simulink model "STEMOLITION_V4_TWOARMCLAW_V1"  (R2021a)
settings: Solver=FixedStepAuto  StartTime=0.0  StopTime=inf  RelTol=1e-3
libraries: vexarmcortexlib x25, vexcommonlib x7
settings Model: ExtModeTrigDuration=25  Creator=nicoa  LastModifiedBy=Mihai Nicoara
settings SolverCC: AlgebraicLoopSolver=TrustRegion
settings OptimizationCC: EnhancedBackFolding=on  PassReuseOutputArgsAs=Individual arguments  ZeroExternalMemoryAtStartup=off  ZeroInternalMemoryAtStartup=off  MaxStackSize=64  OptimizeBlockOrder=speed  DifferentSizesBufferReuse=on  OptimizationCustomize=off  EfficientTunableParamExpr=on
settings DebuggingCC: ParameterTunabilityLossMsg=error  SFMachineParentedDataDiag=warning
settings HardwareCC: ProdBitPerPointer=32  ProdBitPerSizeT=32  ProdBitPerPtrDiffT=32  ProdLargestAtomicInteger=Long  ProdLargestAtomicFloat=Double  ProdWordSize=32  ProdHWDeviceType=ARM Compatible->ARM Cortex
settings SFSimCC: MATLABDynamicMemAlloc=off
settings RTWCC: SystemTargetFile=ert.tlc  HardwareBoard=ARM Cortex-based VEX Microcontroller  TLCOptions="-aInlineSetEventsForThisBaseRateFcn=TLC_FALSE -aSuppressMultiTaskScheduler=TLC_FALSE  -aRateBasedStepFcn=0"  TemplateMakefile=ert_default_tmf  GenerateReport=on  Toolchain=GNU Tools for VEX ARM Cortex  IncludeHyperlinkInReport=on  LaunchReport=on  GenerateTraceInfo=on  GenerateTraceReport=on  GenerateTraceReportSl=on  GenerateTraceReportSf=on  GenerateTraceReportEml=on
settings CodeAppCC: ForceParamTrailComments=on  IgnoreCustomStorageClasses=off  OperatorAnnotations=on  SimulinkDataObjDesc=on  SFDataObjDesc=on  InsertBlockDesc=on

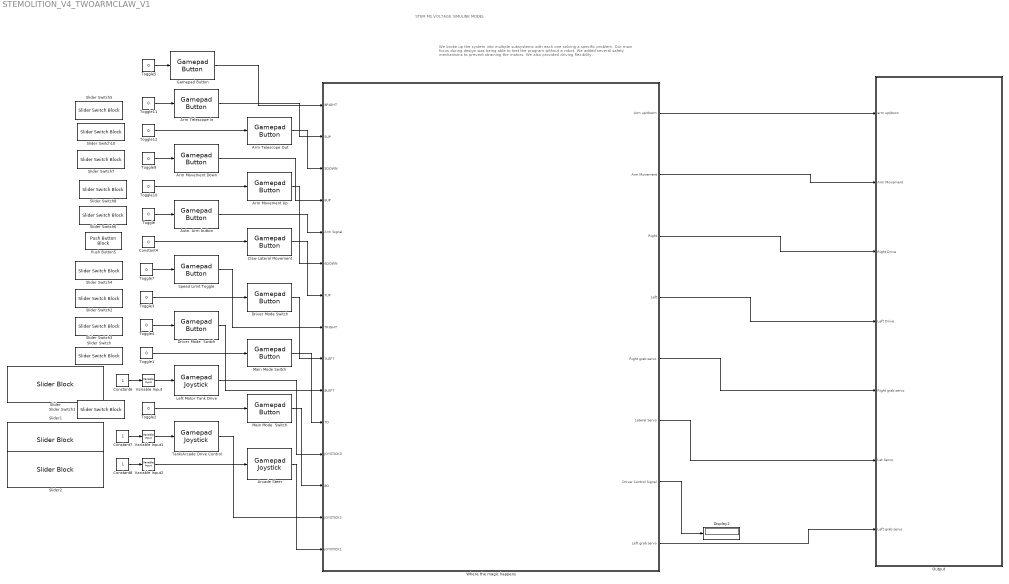
== system STEMOLITION_V4_TWOARMCLAW_V1 ==
  note: We broke up the system into multiple subsystems with each one solving a specific problem. Our main focus during
      | design was being able to test the program without a robot. We added several safety mechanisms to prevent straining
      |  the motors. We also provided driving flexibility.
  note: STEM MS VOLTAGE SIMULINK MODEL
  "Arcade Steer " : vexarmcortexlib/Gamepad/Gamepad Joystick  joystick=1  chan=1  SimulationIn=on  SampleTime=0.02
      settings: SourceProductBaseCode=EC_VEX_MICRO
  Arm Movement Down : vexarmcortexlib/Gamepad/Gamepad Button  joystick=1  chan=6  button56=Down  button78=Down  SimulationIn=on  SampleTime=0.02
      settings: SourceProductBaseCode=EC_VEX_MICRO
  Arm Movement Up : vexarmcortexlib/Gamepad/Gamepad Button  joystick=1  chan=6  button56=Up  button78=Down  SimulationIn=on  SampleTime=0.02
      settings: SourceProductBaseCode=EC_VEX_MICRO
  Arm Telescope In : vexarmcortexlib/Gamepad/Gamepad Button  joystick=1  chan=5  button56=Down  button78=Down  SimulationIn=on  SampleTime=0.02
      settings: SourceProductBaseCode=EC_VEX_MICRO
  Arm Telescope Out : vexarmcortexlib/Gamepad/Gamepad Button  joystick=1  chan=5  button56=Up  button78=Down  SimulationIn=on  SampleTime=0.02
      settings: SourceProductBaseCode=EC_VEX_MICRO
  Auto. Arm button : vexarmcortexlib/Gamepad/Gamepad Button  joystick=1  chan=8  button56=Up  button78=Up  SimulationIn=on  SampleTime=0.02
      settings: SourceProductBaseCode=EC_VEX_MICRO
  Claw Lateral Movement : vexarmcortexlib/Gamepad/Gamepad Button  joystick=1  chan=7  button56=Up  button78=Up  SimulationIn=on  SampleTime=0.02
      settings: SourceProductBaseCode=EC_VEX_MICRO
  Constant4 : Constant  Value=0
  Constant6 : Constant
  Constant7 : Constant
  Constant8 : Constant
  Display2 : Display
  Driver Mode  Switch : vexarmcortexlib/Gamepad/Gamepad Button  joystick=1  chan=8  button56=Up  button78=Left  SimulationIn=on  SampleTime=0.02
      settings: SourceProductBaseCode=EC_VEX_MICRO
  Driver Mode Switch : vexarmcortexlib/Gamepad/Gamepad Button  joystick=1  chan=7  button56=Up  button78=Left  SimulationIn=on  SampleTime=0.02
      settings: SourceProductBaseCode=EC_VEX_MICRO
  Gamepad Button : vexarmcortexlib/Gamepad/Gamepad Button  joystick=1  chan=8  button56=Up  button78=Right  SimulationIn=on  SampleTime=0.02
      settings: SourceProductBaseCode=EC_VEX_MICRO
  Left Motor Tank Drive : vexarmcortexlib/Gamepad/Gamepad Joystick  joystick=1  chan=3  SimulationIn=on  SampleTime=0.02
      settings: SourceProductBaseCode=EC_VEX_MICRO
  Main Mode  Switch : vexarmcortexlib/Gamepad/Gamepad Button  joystick=1  chan=8  button56=Up  button78=Down  SimulationIn=on  SampleTime=0.02
      settings: SourceProductBaseCode=EC_VEX_MICRO
  Main Mode Switch : vexarmcortexlib/Gamepad/Gamepad Button  joystick=1  chan=7  button56=Up  button78=Down  SimulationIn=on  SampleTime=0.02
      settings: SourceProductBaseCode=EC_VEX_MICRO
  Output : Subsystem
  Push Button5 : PushButtonBlock
  Slider : SliderBlock  LabelPosition=Hide  ScaleMin=-127  ScaleMax=127
  Slider Switch{,1..5,7..8,10} (9 alike) : SliderSwitchBlock  LabelPosition=Hide
      settings: Values={{'Off', 'On'}, [0 1]}
  Slider Switch6 : SliderSwitchBlock
      settings: Values={{'Off', 'On'}, [0 1]}
  Slider1 : SliderBlock  LabelPosition=Hide  ScaleMin=-127  ScaleMax=127
  Slider2 : SliderBlock  LabelPosition=Hide  ScaleMin=-127  ScaleMax=127
  Speed Limit Toggle : vexarmcortexlib/Gamepad/Gamepad Button  joystick=1  chan=7  button56=Up  button78=Right  SimulationIn=on  SampleTime=0.02
      settings: SourceProductBaseCode=EC_VEX_MICRO
  Tank/Arcade Drive Control : vexarmcortexlib/Gamepad/Gamepad Joystick  joystick=1  chan=2  SimulationIn=on  SampleTime=0.02
      settings: SourceProductBaseCode=EC_VEX_MICRO
  Toggle{,1..5,7,9..12} (11 alike) : Constant  Value=0
      settings: OpenFcn=|
      | if strcmp('0',get_param(gcb, 'Value'))                        set_param(gcb, 'Value', '1');
      | else
      |             set_param(gcb, 'Value', '0');
      | end
  Variable Input : vexarmcortexlib/Utilities/Variable Input  low=-127  gain=-29.69085144927537  high=127
      settings: SourceProductBaseCode=EC_VEX_MICRO
  Variable Input1 : vexarmcortexlib/Utilities/Variable Input  low=-127  gain=0  high=127
      settings: SourceProductBaseCode=EC_VEX_MICRO
  Variable Input2 : vexarmcortexlib/Utilities/Variable Input  low=-127  gain=0  high=127
      settings: SourceProductBaseCode=EC_VEX_MICRO
  Where the magic happens : Subsystem
  wires:
  Main Mode  Switch/1 -> Where the magic happens/13(8D)
  Main Mode Switch/1 -> Where the magic happens/11(7D)
  Driver Mode  Switch/1 -> Where the magic happens/10(8LEFT)
  Driver Mode Switch/1 -> Where the magic happens/9(7LEFT)
  Speed Limit Toggle/1 -> Where the magic happens/8(7RIGHT)
  Tank/Arcade Drive Control/1 -> Where the magic happens/14(JOYSTICK2)
  Left Motor Tank Drive/1 -> Where the magic happens/12(JOYSTICK3)
  "Arcade Steer "/1 -> Where the magic happens/15(JOYSTICK1)
  Claw Lateral Movement/1 -> Where the magic happens/7(7UP)
  Arm Movement Up/1 -> Where the magic happens/6(6DOWN)
  Arm Movement Down/1 -> Where the magic happens/4(6UP)
  Arm Telescope Out/1 -> Where the magic happens/3(5DOWN)
  Arm Telescope In/1 -> Where the magic happens/2(5UP)
  Toggle11/1 -> Arm Telescope In/1
  Toggle12/1 -> Arm Telescope Out/1
  Toggle9/1 -> Arm Movement Down/1
  Toggle10/1 -> Arm Movement Up/1
  Constant4/1 -> Claw Lateral Movement/1
  Toggle7/1 -> Speed Limit Toggle/1
  Toggle4/1 -> Driver Mode  Switch/1
  Toggle1/1 -> Main Mode Switch/1
  Constant6/1 -> Variable Input/1
  Variable Input/1 -> Left Motor Tank Drive/1
  Variable Input1/1 -> Tank/Arcade Drive Control/1
  Constant7/1 -> Variable Input1/1
  Variable Input2/1 -> "Arcade Steer "/1
  Constant8/1 -> Variable Input2/1
  Toggle2/1 -> Main Mode  Switch/1
  Toggle3/1 -> Driver Mode Switch/1
  Where the magic happens/7(Driver Control Signal) -> Display2/1
  Where the magic happens/6(Lateral Servo) -> Output/6(Lat Servo)
  Where the magic happens/5(Right grab servo) -> Output/5(Right grab servo)
  Where the magic happens/1(Arm up/dowm) -> Output/1(arm up/down)
  Where the magic happens/2(Arm Movement) -> Output/2(Arm Movement)
  Toggle5/1 -> Gamepad Button/1
  Gamepad Button/1 -> Where the magic happens/1(8RIGHT)
  Where the magic happens/3(Right) -> Output/3(Right Drive)
  Where the magic happens/4(Left) -> Output/4(Left Drive)
  Auto. Arm button/1 -> Where the magic happens/5(Arm Signal)
  Toggle/1 -> Auto. Arm button/1
  Where the magic happens/8(Left grab servo) -> Output/7(Left grab servo)

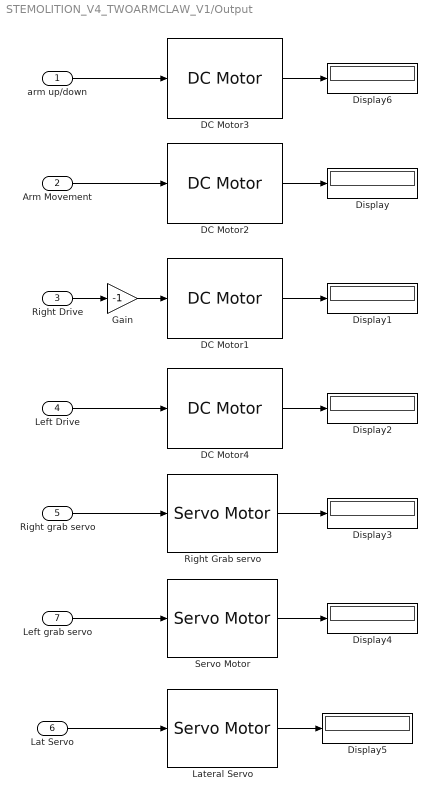
== system STEMOLITION_V4_TWOARMCLAW_V1/Output ==
  arm up/down : Inport
  Arm Movement : Inport  Port=2
  Right Drive : Inport  Port=3
  Left Drive : Inport  Port=4
  Right grab servo : Inport  Port=5
  Lat Servo : Inport  Port=6
  Left grab servo : Inport  Port=7
  DC Motor1 : vexarmcortexlib/Actuators/DC Motor  motor=2  scaleFactor=1/13.5  SimulationOut=on
      settings: SourceProductBaseCode=EC_VEX_MICRO
  DC Motor2 : vexarmcortexlib/Actuators/DC Motor  motor=4  scaleFactor=1/13.5  SimulationOut=on
      settings: SourceProductBaseCode=EC_VEX_MICRO
  DC Motor3 : vexarmcortexlib/Actuators/DC Motor  motor=7  scaleFactor=1/13.5  SimulationOut=on
      settings: SourceProductBaseCode=EC_VEX_MICRO
  DC Motor4 : vexarmcortexlib/Actuators/DC Motor  motor=9  scaleFactor=1/13.5  SimulationOut=on
      settings: SourceProductBaseCode=EC_VEX_MICRO
  Display{,1..6} (7 alike) : Display
  Gain : Gain  Gain=-1
  Lateral Servo : vexarmcortexlib/Actuators/Servo Motor  motor=8  scaleFactor=60/127  SimulationOut=on
      settings: SourceProductBaseCode=EC_VEX_MICRO
  Right Grab servo : vexarmcortexlib/Actuators/Servo Motor  motor=3  scaleFactor=60/127  SimulationOut=on
      settings: SourceProductBaseCode=EC_VEX_MICRO
  Servo Motor : vexarmcortexlib/Actuators/Servo Motor  motor=5  scaleFactor=60/127  SimulationOut=on
      settings: SourceProductBaseCode=EC_VEX_MICRO
  wires:
  Right Grab servo/1 -> Display3/1
  Arm Movement/1 -> DC Motor2/1
  Right grab servo/1 -> Right Grab servo/1
  DC Motor2/1 -> Display/1
  DC Motor3/1 -> Display6/1
  DC Motor4/1 -> Display2/1
  DC Motor1/1 -> Display1/1
  Lateral Servo/1 -> Display5/1
  arm up/down/1 -> DC Motor3/1
  Lat Servo/1 -> Lateral Servo/1
  Right Drive/1 -> Gain/1
  Left Drive/1 -> DC Motor4/1
  Gain/1 -> DC Motor1/1
  Servo Motor/1 -> Display4/1
  Left grab servo/1 -> Servo Motor/1

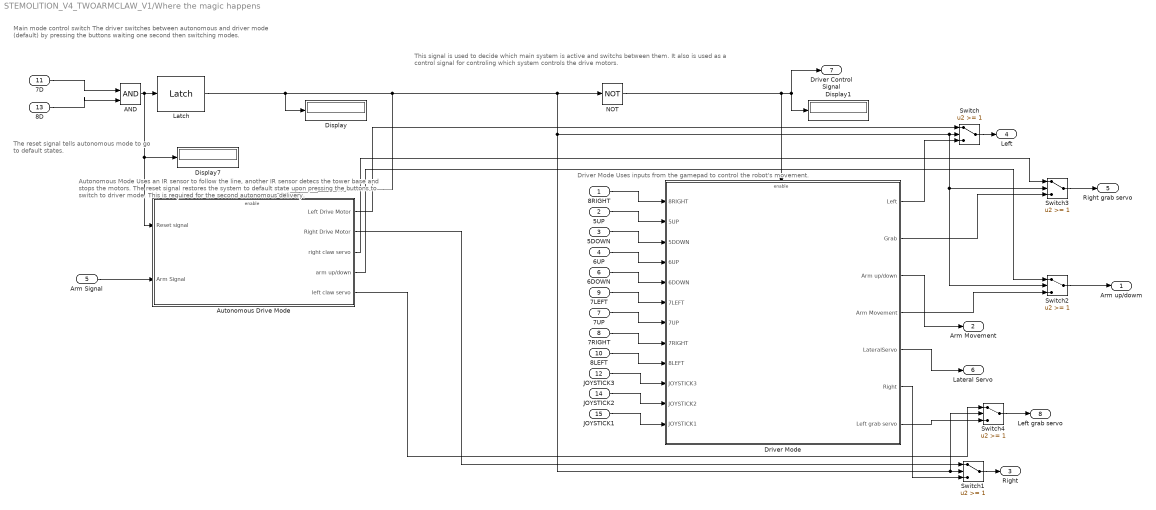
== system STEMOLITION_V4_TWOARMCLAW_V1/Where the magic happens ==
  note: Driver Mode
      | Uses inputs from the gamepad to control the robot's movement.
  note: This signal is used to decide which main system is active and switchs between them.
      | It also is used as a control signal for controling which system controls the drive motors.
  note: The reset signal tells autonomous
      | mode to go to default states.
  note: Autonomous Mode
      | 	Uses an IR sensor to follow the line, another IR sensor detecs the
      | 	tower base and stops the motors. The reset signal restores the system
      | 	to default state upon pressing the buttons to switch to driver mode. This
      | 	is required for the second autonomous delivery.
  note: Main mode control switch
      | The driver switches between autonomous and driver mode (default) by
      | pressing the buttons waiting one second then switching modes.
  8RIGHT : Inport
  5UP : Inport  Port=2
  5DOWN : Inport  Port=3
  6UP : Inport  Port=4
  Arm Signal : Inport  Port=5
  6DOWN : Inport  Port=6
  7UP : Inport  Port=7
  7RIGHT : Inport  Port=8
  7LEFT : Inport  Port=9
  8LEFT : Inport  Port=10
  7D : Inport  Port=11
  JOYSTICK3 : Inport  Port=12
  8D : Inport  Port=13
  JOYSTICK2 : Inport  Port=14
  JOYSTICK1 : Inport  Port=15
  "AND " : Logic  IconShape=distinctive  AllPortsSameDT=off  OutDataTypeStr=boolean
  Autonomous Drive Mode : Subsystem
  Display : Display
  Display1 : Display
  Display7 : Display
  Driver Mode : Subsystem  TreatAsAtomicUnit=on
  Latch : vexcommonlib/Latch  output0=off  BlockPlatform=vexarmcortex
      settings: SourceProductBaseCode=EC_VEX_MICRO,VEXV5
  NOT : Logic  Operator=NOT  IconShape=distinctive  AllPortsSameDT=off  OutDataTypeStr=boolean
  Switch{,1..4} (5 alike) : Switch  Threshold=1
  Arm up/dowm : Outport
  Arm Movement : Outport  Port=2
  Right : Outport  Port=3
  Left : Outport  Port=4
  Right grab servo : Outport  Port=5
  Lateral Servo : Outport  Port=6
  Driver Control Signal : Outport  Port=7
  Left grab servo : Outport  Port=8
  wires:
  7D/1 -> "AND "/1
  "AND "/1 -> Latch/1, Display7/1, Autonomous Drive Mode/1(Reset signal)
  8D/1 -> "AND "/2
  Latch/1 -> Display/1, Autonomous Drive Mode/Enable, NOT/1, Switch4/2, Switch1/2, Switch3/2, Switch2/2, Switch/2
  NOT/1 -> Driver Mode/Enable, Display1/1, Driver Control Signal/1
  Autonomous Drive Mode/1(Left Drive Motor) -> Switch/1
  Switch/1 -> Left/1
  Autonomous Drive Mode/2(Right Drive Motor) -> Switch1/1
  Switch1/1 -> Right/1
  Switch2/1 -> Arm up/dowm/1
  Autonomous Drive Mode/4(arm up/down) -> Switch2/1
  Switch3/1 -> Right grab servo/1
  Autonomous Drive Mode/3(right claw servo) -> Switch3/1
  Arm Signal/1 -> Autonomous Drive Mode/2(Arm Signal)
  JOYSTICK1/1 -> Driver Mode/12(JOYSTICK1)
  JOYSTICK2/1 -> Driver Mode/11(JOYSTICK2)
  JOYSTICK3/1 -> Driver Mode/10(JOYSTICK3)
  8LEFT/1 -> Driver Mode/9(8LEFT)
  7RIGHT/1 -> Driver Mode/8(7RIGHT)
  7UP/1 -> Driver Mode/7(7UP)
  7LEFT/1 -> Driver Mode/6(7LEFT)
  6DOWN/1 -> Driver Mode/5(6DOWN)
  6UP/1 -> Driver Mode/4(6UP)
  5DOWN/1 -> Driver Mode/3(5DOWN)
  5UP/1 -> Driver Mode/2(5UP)
  8RIGHT/1 -> Driver Mode/1(8RIGHT)
  Driver Mode/1(Left) -> Switch/3
  Driver Mode/5(LateralServo) -> Lateral Servo/1
  Driver Mode/6(Right) -> Switch1/3
  Driver Mode/4(Arm Movement) -> Switch2/3
  Driver Mode/3(Arm up/down) -> Arm Movement/1
  Driver Mode/2(Grab) -> Switch3/3
  Switch4/1 -> Left grab servo/1
  Autonomous Drive Mode/5(left claw servo) -> Switch4/1
  Driver Mode/7(Left grab servo) -> Switch4/3

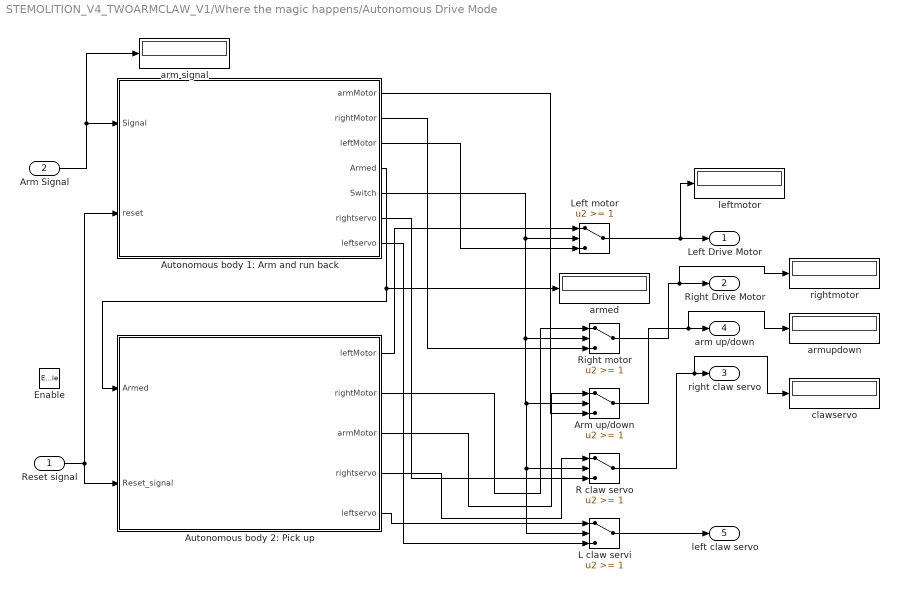
== system STEMOLITION_V4_TWOARMCLAW_V1/Where the magic happens/Autonomous Drive Mode ==
  Reset signal : Inport
  Arm Signal : Inport  Port=2
  Enable : EnablePort  StatesWhenEnabling=reset
  Arm up/down : Switch  Threshold=1
  Autonomous body 1: Arm and run back : Stateflow chart  TreatAsAtomicUnit=on
  Autonomous body 2: Pick up : Stateflow chart  TreatAsAtomicUnit=on
  L claw servi : Switch  Threshold=1
  Left motor : Switch  Threshold=1
  R claw servo : Switch  Threshold=1
  Right motor : Switch  Threshold=1
  arm signal : Display
  armed : Display
  armupdown : Display
  clawservo : Display
  leftmotor : Display
  rightmotor : Display
  Left Drive Motor : Outport
  Right Drive Motor : Outport  Port=2
  right claw servo : Outport  Port=3
  arm up/down : Outport  Port=4
  left claw servo : Outport  Port=5
  wires:
  Reset signal/1 -> Autonomous body 1: Arm and run back/2(reset), Autonomous body 2: Pick up/2(Reset_signal)
  Arm Signal/1 -> arm signal/1, Autonomous body 1: Arm and run back/1(Signal)
  Autonomous body 1: Arm and run back/4(Armed) -> armed/1, Autonomous body 2: Pick up/1(Armed)
  Left motor/1 -> leftmotor/1, Left Drive Motor/1
  Right motor/1 -> rightmotor/1, Right Drive Motor/1
  Arm up/down/1 -> armupdown/1, arm up/down/1
  R claw servo/1 -> clawservo/1, right claw servo/1
  Autonomous body 2: Pick up/1(leftMotor) -> Left motor/1
  Autonomous body 1: Arm and run back/5(Switch) -> L claw servi/2, R claw servo/2, Arm up/down/2, Right motor/2, Left motor/2
  Autonomous body 2: Pick up/2(rightMotor) -> Right motor/1
  Autonomous body 2: Pick up/3(armMotor) -> Arm up/down/1
  Autonomous body 1: Arm and run back/3(leftMotor) -> Left motor/3
  Autonomous body 1: Arm and run back/2(rightMotor) -> Right motor/3
  Autonomous body 1: Arm and run back/1(armMotor) -> Arm up/down/3
  Autonomous body 1: Arm and run back/6(rightservo) -> R claw servo/3
  L claw servi/1 -> left claw servo/1
  Autonomous body 1: Arm and run back/7(leftservo) -> L claw servi/3
  Autonomous body 2: Pick up/4(rightservo) -> R claw servo/1
  Autonomous body 2: Pick up/5(leftservo) -> L claw servi/1

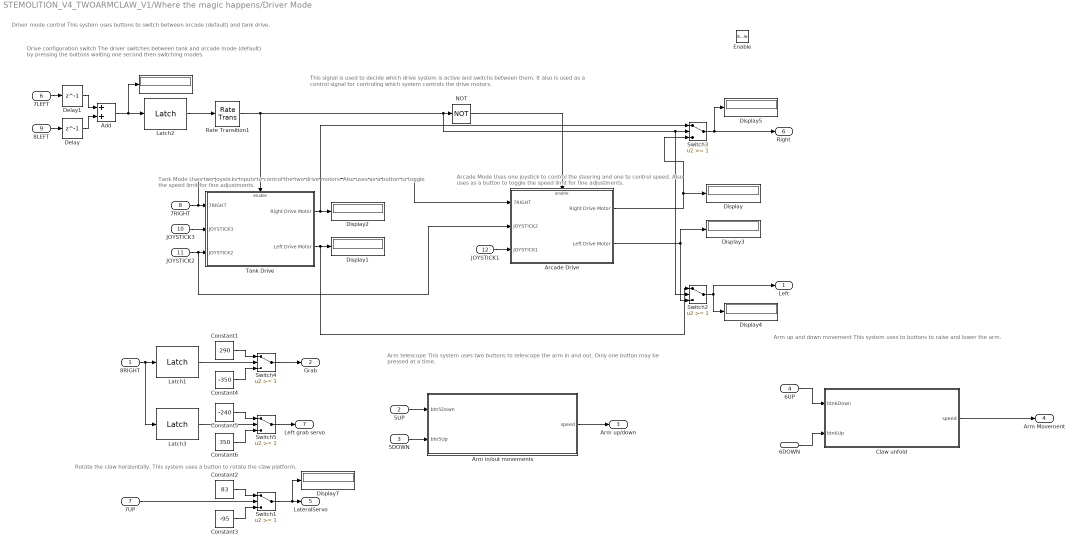
== system STEMOLITION_V4_TWOARMCLAW_V1/Where the magic happens/Driver Mode ==
  note: Tank Mode
      | Uses two joysticks inputs to control the two drive motors. Also uses as a button
      | to toggle the speed limit for fine adjustments.
  note: Arm up and down movement
      | This system uses to buttons to raise and lower the arm.
  note: Drive configuration switch
      | The driver switches between tank and arcade mode (default) by
      | pressing the buttons waiting one second then switching modes.
  note: Rotate the claw horizontally.
      | This system uses a button to rotate the claw platform.
  note: Arm telescope
      | This system uses two buttons to telescope the arm in and out.
      | Only one button may be pressed at a time.
  note: Driver mode control
      | This system uses buttons to switch between arcade (default) and tank drive.
  note: This signal is used to decide which drive system is active and switchs between them.
      | It also is used as a control signal for controling which system controls the drive motors.
  note: Arcade Mode
      | Uses one joystick to control the steering and one to control  speed.
      | Also uses as a button to toggle the speed limit for fine  adjustments.
  8RIGHT : Inport
  5UP : Inport  Port=2
  5DOWN : Inport  Port=3
  6UP : Inport  Port=4
  6DOWN : Inport  Port=5
  7LEFT : Inport  Port=6
  7UP : Inport  Port=7
  7RIGHT : Inport  Port=8
  8LEFT : Inport  Port=9
  JOYSTICK3 : Inport  Port=10
  JOYSTICK2 : Inport  Port=11
  JOYSTICK1 : Inport  Port=12
  Enable : EnablePort
  " " : Display
  Add : Sum
  "Arcade Drive " : Subsystem  TreatAsAtomicUnit=on
  Arm in/out movements : Stateflow chart  TreatAsAtomicUnit=on
  Claw unfold : Stateflow chart  TreatAsAtomicUnit=on
  Constant1 : Constant  Value=290
  Constant2 : Constant  Value=83
  Constant3 : Constant  Value=-95
  Constant4 : Constant  Value=-350
  Constant5 : Constant  Value=-240
  Constant6 : Constant  Value=350
  Delay : Delay  DelayLength=1  InitialCondition=0  SampleTime=0.5
  Delay1 : Delay  DelayLength=1  InitialCondition=0  SampleTime=0.5
  Display{,1..5,7} (7 alike) : Display
  Latch1 : vexcommonlib/Latch  output0=off  BlockPlatform=vexarmcortex
      settings: SourceProductBaseCode=EC_VEX_MICRO,VEXV5
  Latch2 : vexcommonlib/Latch  output0=off  BlockPlatform=vexarmcortex
      settings: SourceProductBaseCode=EC_VEX_MICRO,VEXV5
  Latch3 : vexcommonlib/Latch  output0=off  BlockPlatform=vexarmcortex
      settings: SourceProductBaseCode=EC_VEX_MICRO,VEXV5
  NOT : Logic  Operator=NOT  IconShape=distinctive  AllPortsSameDT=off  OutDataTypeStr=boolean
  Rate Transition1 : RateTransition  OutPortSampleTime=0.002
  Switch{1..5} (5 alike) : Switch  Threshold=1
  "Tank Drive " : Subsystem  TreatAsAtomicUnit=on
  Left : Outport
  Grab : Outport  Port=2
  Arm up/down : Outport  Port=3
  Arm Movement : Outport  Port=4
  LateralServo : Outport  Port=5
  Right : Outport  Port=6
  Left grab servo : Outport  Port=7
  wires:
  Constant6/1 -> Switch5/3
  Latch3/1 -> Switch5/2
  Constant5/1 -> Switch5/1
  Constant1/1 -> Switch4/1
  Claw unfold/1(speed) -> Arm Movement/1
  5UP/1 -> Arm in/out movements/1(btn5Down)
  Switch4/1 -> Grab/1
  5DOWN/1 -> Arm in/out movements/2(btn5Up)
  "Tank Drive "/2(Left Drive Motor) -> Display1/1, Switch2/1
  Switch3/1 -> Right/1, Display5/1
  JOYSTICK1/1 -> "Arcade Drive "/3(JOYSTICK1)
  "Arcade Drive "/1(Right Drive Motor) -> Display/1, Switch3/3
  8RIGHT/1 -> Latch3/1, Latch1/1
  "Tank Drive "/1(Right Drive Motor) -> Display2/1, Switch3/1
  7LEFT/1 -> Delay1/1
  7RIGHT/1 -> "Tank Drive "/1(7RIGHT), "Arcade Drive "/1(7RIGHT)
  "Arcade Drive "/2(Left Drive Motor) -> Switch2/3, Display3/1
  Constant3/1 -> Switch1/3
  Constant2/1 -> Switch1/1
  NOT/1 -> "Arcade Drive "/Enable
  Switch5/1 -> Left grab servo/1
  7UP/1 -> Switch1/2
  Add/1 -> " "/1, Latch2/1
  JOYSTICK2/1 -> "Tank Drive "/3(JOYSTICK2), "Arcade Drive "/2(JOYSTICK2)
  Latch1/1 -> Switch4/2
  JOYSTICK3/1 -> "Tank Drive "/2(JOYSTICK3)
  Switch1/1 -> Display7/1, LateralServo/1
  8LEFT/1 -> Delay/1
  Delay/1 -> Add/2
  Arm in/out movements/1(speed) -> Arm up/down/1
  Latch2/1 -> Rate Transition1/1
  Rate Transition1/1 -> NOT/1, Switch2/2, Switch3/2, "Tank Drive "/Enable
  Constant4/1 -> Switch4/3
  Switch2/1 -> Display4/1, Left/1
  Delay1/1 -> Add/1
  6UP/1 -> Claw unfold/1(btn6Down)
  6DOWN/1 -> Claw unfold/2(btn6Up)

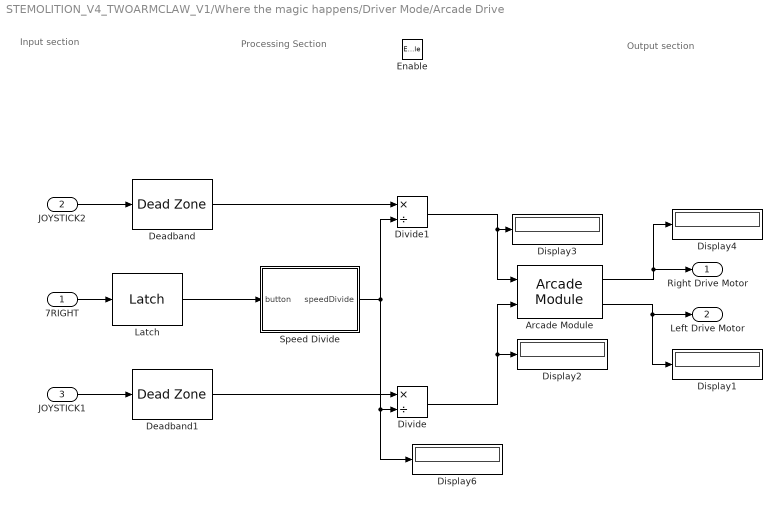
== system STEMOLITION_V4_TWOARMCLAW_V1/Where the magic happens/Driver Mode/Arcade Drive  ==
  note: Output section
  note: Processing Section
  note: Input section
  7RIGHT : Inport
  JOYSTICK2 : Inport  Port=2
  JOYSTICK1 : Inport  Port=3
  Enable : EnablePort
  Arcade Module : vexcommonlib/Arcade Module  BlockPlatform=vexarmcortex
      settings: SourceProductBaseCode=EC_VEX_MICRO,VEXV5
  Deadband : DeadZone  LowerValue=-9  UpperValue=9  SaturateOnIntegerOverflow=on
  Deadband1 : DeadZone  LowerValue=-9  UpperValue=9  SaturateOnIntegerOverflow=on
  Display{1..4,6} (5 alike) : Display
  Divide : Product  Inputs=*/
  Divide1 : Product  Inputs=*/
  Latch : vexcommonlib/Latch  output0=off  BlockPlatform=vexarmcortex
      settings: SourceProductBaseCode=EC_VEX_MICRO,VEXV5
  Speed Divide : Stateflow chart  TreatAsAtomicUnit=on
  Right Drive Motor : Outport
  Left Drive Motor : Outport  Port=2
  wires:
  7RIGHT/1 -> Latch/1
  Speed Divide/1(speedDivide) -> Display6/1, Divide/2, Divide1/2
  Divide/1 -> Arcade Module/2, Display2/1
  Divide1/1 -> Arcade Module/1, Display3/1
  Arcade Module/1 -> Display4/1, Right Drive Motor/1
  Arcade Module/2 -> Display1/1, Left Drive Motor/1
  Latch/1 -> Speed Divide/1(button)
  JOYSTICK2/1 -> Deadband/1
  JOYSTICK1/1 -> Deadband1/1
  Deadband/1 -> Divide1/1
  Deadband1/1 -> Divide/1

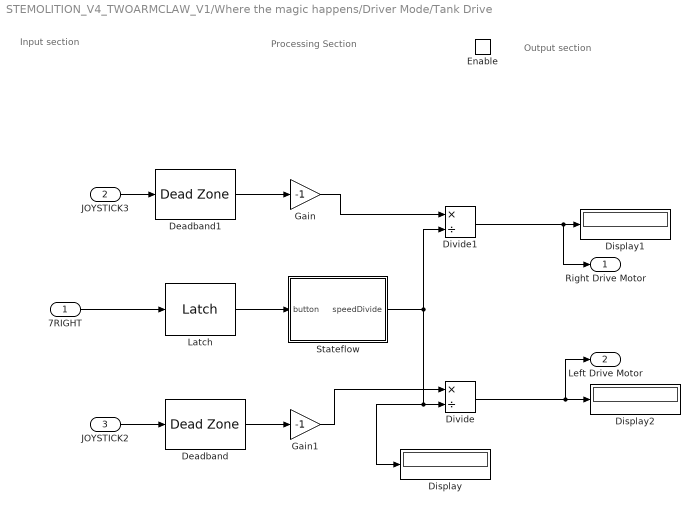
== system STEMOLITION_V4_TWOARMCLAW_V1/Where the magic happens/Driver Mode/Tank Drive  ==
  note: Output section
  note: Processing Section
  note: Input section
  7RIGHT : Inport
  JOYSTICK3 : Inport  Port=2
  JOYSTICK2 : Inport  Port=3
  Enable : EnablePort
  Deadband : DeadZone  LowerValue=-9  UpperValue=9  SaturateOnIntegerOverflow=on
  Deadband1 : DeadZone  LowerValue=-9  UpperValue=9  SaturateOnIntegerOverflow=on
  Display : Display
  Display1 : Display
  Display2 : Display
  Divide : Product  Inputs=*/
  Divide1 : Product  Inputs=*/
  Gain : Gain  Gain=-1
  Gain1 : Gain  Gain=-1
  Latch : vexcommonlib/Latch  output0=off  BlockPlatform=vexarmcortex
      settings: SourceProductBaseCode=EC_VEX_MICRO,VEXV5
  Stateflow : Stateflow chart  TreatAsAtomicUnit=on
  Right Drive Motor : Outport
  Left Drive Motor : Outport  Port=2
  wires:
  7RIGHT/1 -> Latch/1
  Latch/1 -> Stateflow/1(button)
  Stateflow/1(speedDivide) -> Divide1/2, Display/1, Divide/2
  JOYSTICK3/1 -> Deadband1/1
  Divide1/1 -> Display1/1, Right Drive Motor/1
  Divide/1 -> Display2/1, Left Drive Motor/1
  JOYSTICK2/1 -> Deadband/1
  Gain/1 -> Divide1/1
  Gain1/1 -> Divide/1
  Deadband1/1 -> Gain/1
  Deadband/1 -> Gain1/1

== stateflow chart STEMOLITION_V4_TWOARMCLAW_V1/Where the magic happens/Driver Mode/Arm in//out movements ==
  state ARMDOWN
    entry:
    speed = -80;
  state STOPPED
    entry:
    speed = 0;
  state ARMUP
    entry:
    speed = 80;
  (default) -> STOPPED
  STOPPED -> ARMUP [order 1] : [btn5Down == 0 && btn5Up == 1 ]
  STOPPED -> ARMDOWN [order 2] : [btn5Down == 1 && btn5Up == 0]
  ARMDOWN -> STOPPED [order 2] : [btn5Down == 0]
  ARMUP -> STOPPED [order 2] : [btn5Up == 0]
  ARMDOWN -> STOPPED [order 1] : [btn5Down == 1 && btn5Up == 1]
  ARMUP -> STOPPED [order 1] : [btn5Down == 1 && btn5Up == 1]
  data: btn5Down input; btn5Up input; speed output

== stateflow chart STEMOLITION_V4_TWOARMCLAW_V1/Where the magic happens/Driver Mode/Claw unfold ==
  state ARMDOWN
    entry:
    speed = -50;
  state STOPPED
    entry:
    speed = 0;
  state ARMUP
    entry:
    speed = 140;
  (default) -> STOPPED
  STOPPED -> ARMUP [order 1] : [btn6Down == 0 && btn6Up == 1 ]
  STOPPED -> ARMDOWN [order 2] : [btn6Down == 1 && btn6Up == 0]
  ARMDOWN -> STOPPED [order 2] : [btn6Down == 0]
  ARMUP -> STOPPED [order 2] : [btn6Up == 0]
  ARMDOWN -> STOPPED [order 1] : [btn6Down == 1 && btn6Up == 1]
  ARMUP -> STOPPED [order 1] : [btn6Down == 1 && btn6Up == 1]
  data: speed output; btn6Down input; btn6Up input

== stateflow chart STEMOLITION_V4_TWOARMCLAW_V1/Where the magic happens/Autonomous Drive Mode/Autonomous body 2: Pick up ==
  state Echo
    entry:
    leftMotor = 0;
    rightMotor = 0;
    armMotor = -60;
  state Armed
    entry:
    leftMotor = 0;
    rightMotor = 0;
    armMotor = 0;
  state Charlie
    entry:
    leftMotor = 0;
    rightMotor = 0;
    armMotor = 0;
  state Delta
    entry:
    leftMotor = -90;
    rightMotor = -90;
    armMotor = 0;
  state Foxtrot
    entry:
    leftMotor = 0;
    rightMotor = 0;
    armMotor =  0;
    rightservo = 200;
    leftservo = -200;
  state Golf
    entry:
    leftMotor = 0;
    rightMotor = 0;
    armMotor =  40;
    rightservo = 200;
    leftservo = -200;
  state Hotel
    entry:
    leftMotor = 115;
    rightMotor = 115;
    armMotor =  0;
    rightservo = 200;
    leftservo = -200;
  state India
    entry:
    leftMotor = 0;
    rightMotor = 0;
    armMotor =  0;
    rightservo = 200;
    leftservo = -200;
  (default) -> Armed
  India -> Armed : [Reset_signal == 1]
  Armed -> Charlie : [Armed == 1]
  Charlie -> Delta : [after(2.5,sec)]
  Delta -> Echo : [after(1.3,sec)]
  Echo -> Foxtrot : [after(1,sec)]
  Foxtrot -> Golf : [after(1,sec)]
  Golf -> Hotel : [after(0.8, sec)]
  Hotel -> India : [after(1.7,sec)]
  data: Armed input; leftMotor output; rightMotor output; armMotor output; Reset_signal input; rightservo output; leftservo output

== stateflow chart STEMOLITION_V4_TWOARMCLAW_V1/Where the magic happens/Autonomous Drive Mode/Autonomous body 1: Arm and run back ==
  state Pre_Armed
    entry:
    leftMotor = 0;
    rightMotor = 0;
    armMotor = 0;
    Armed = 0;
    Switch = 0;
  state Alfa
    entry:
    leftMotor = 0;
    rightMotor = 0;
    armMotor = 50;
    rightservo = -350;
    leftservo = 350;
    Armed = 0;
  state Bravo
    entry:
    leftMotor = 130;
    rightMotor = 130;
    armMotor = 0;
    Armed = 0;
  state ARMED
    entry:
    Armed = 1;
    Switch = 1;
  state Start
    entry:
    leftMotor = 0;
    rightMotor = 0;
    armMotor = 0;
    rightservo = -350;
    leftservo = 350;
    Armed = 0;
  Pre_Armed -> ARMED : [Signal == 1]
  (default) -> Start
  Alfa -> Bravo : [after(1.3,sec)]
  Start -> Alfa : [after(2,sec)]
  ARMED -> Start : [reset == 1]
  Bravo -> Pre_Armed : [after(1.3,sec)]
  data: armMotor output; rightMotor output; leftMotor output; Signal input; Armed output; reset input; Switch output; rightservo output; leftservo output

== stateflow chart STEMOLITION_V4_TWOARMCLAW_V1/Where the magic happens/Driver Mode/Arcade Drive /Speed Divide ==
  state Full_Speed
    entry:
    speedDivide = 1
  state Slow_Speed
    entry:
    speedDivide = 2
  (default) -> Full_Speed
  Full_Speed -> Slow_Speed : [button == 1]
  Slow_Speed -> Full_Speed : [button == 0]
  data: speedDivide output; button input

== stateflow chart STEMOLITION_V4_TWOARMCLAW_V1/Where the magic happens/Driver Mode/Tank Drive /Stateflow ==
  state Full_Speed
    entry:
    speedDivide = 1
  state Slow_Speed
    entry:
    speedDivide = 2
  (default) -> Full_Speed
  Full_Speed -> Slow_Speed : [button]
  Slow_Speed -> Full_Speed : [button == 0]
  data: speedDivide output; button input
